simulink model "PSV-based Ventilator Circuit"  (R2016a)
settings: Solver=VariableStepAuto  StartTime=0.0  StopTime=10.0  RelTol=1e-3
undefined symbols (not defined in the file): alfa, cdd, cl, fms, kms, mms, PA, PB, Ps, PT, roh
libraries: sh_lib x5, fl_lib x5
settings Model: Creator=sarim  LastModifiedBy=sarim

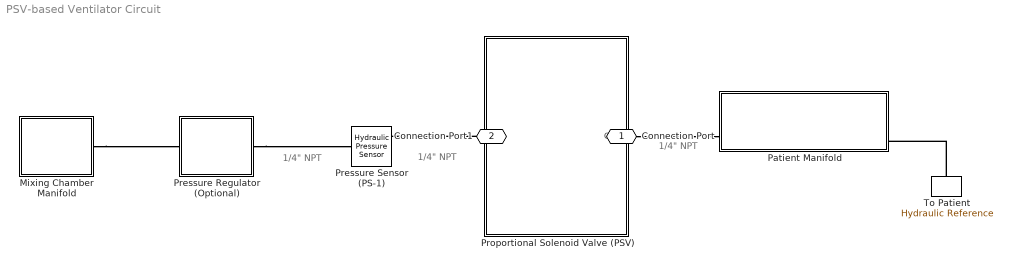
== system PSV-based Ventilator Circuit ==
  note: 1/4" NPT
  note: 1/4" NPT
  note: 1/4" NPT
  Mixing Chamber Manifold : Subsystem
  Patient Manifold : Subsystem
  Pressure Regulator (Optional) : Subsystem
  Pressure Sensor (PS-1) : fl_lib/Hydraulic/Hydraulic Sensors/Hydraulic Pressure Sensor
  Proportional Solenoid Valve (PSV) : Subsystem  VariantControl=Variant1
      mask Display: image('C:\Users\sarim\Desktop\Untitled.png');
  To Patient : fl_lib/Hydraulic/Hydraulic Elements/Hydraulic Reference
  Connection Port : PMIOPort  Port=1  Side=Left
  Connection Port1 : PMIOPort  Port=2  Side=Right
  connections:
  Pressure Regulator (Optional)/RConn1 -- Pressure Sensor (PS-1)/LConn1
  Connection Port1/RConn1 -- Pressure Sensor (PS-1)/RConn1
  Connection Port/RConn1 -- Patient Manifold/LConn2
  To Patient/LConn1 -- Patient Manifold/RConn3
  Mixing Chamber Manifold/RConn1 -- Pressure Regulator (Optional)/LConn1

== system PSV-based Ventilator Circuit/Mixing Chamber Manifold ==
  Air In : PMIOPort  Port=1  Side=Left
  Out : PMIOPort  Port=2  Side=Right
  O2 In : PMIOPort  Port=3  Side=Left

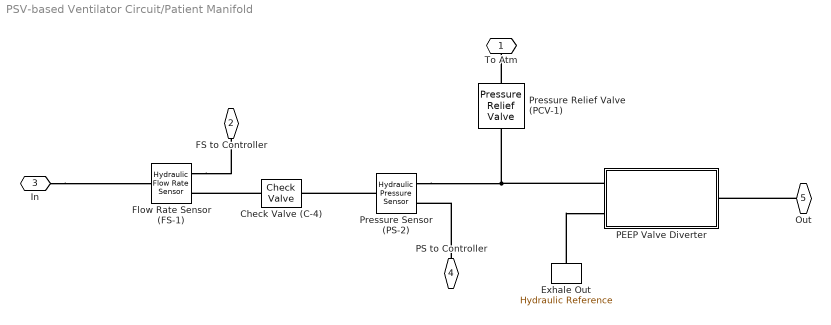
== system PSV-based Ventilator Circuit/Patient Manifold ==
  Check Valve (C-4) : sh_lib/Valves/Directional Valves/Check Valve  area_max=1e-4 m^2  pres_crack=0.3e5 Pa  pres_max=1.2e5 Pa  C_d=0.7  Re_cr=12  A_leak=1e-12 m^2  dynamic=0  tau=0.1 s  area_init=1e-12 m^2
  Exhale Out : fl_lib/Hydraulic/Hydraulic Elements/Hydraulic Reference
  Flow Rate Sensor (FS-1) : fl_lib/Hydraulic/Hydraulic Sensors/Hydraulic Flow Rate Sensor
  PEEP Valve Diverter : Subsystem
  Pressure Sensor (PS-2) : fl_lib/Hydraulic/Hydraulic Sensors/Hydraulic Pressure Sensor
  Pressure Relief Valve (PCV-1) : sh_lib/Valves/Pressure Control Valves/Pressure Relief Valve  area_max=1e-4 m^2  pres_set=50e5 Pa  reg_range=5e5 Pa  C_d=0.7  Re_cr=12  A_leak=1e-12 m^2  dynamic=0  tau=0.1 s  area_init=1e-12 m^2
  To Atm : PMIOPort  Port=1  Side=Left
  FS to Controller : PMIOPort  Port=2  Side=Right
  In : PMIOPort  Port=3  Side=Left
  PS to Controller : PMIOPort  Port=4  Side=Right
  Out : PMIOPort  Port=5  Side=Right
  connections:
  Pressure Relief Valve (PCV-1)/RConn1 -- To Atm/RConn1
  Flow Rate Sensor (FS-1)/RConn1 -- FS to Controller/RConn1
  Exhale Out/LConn1 -- PEEP Valve Diverter/LConn2
  Pressure Sensor (PS-2)/LConn1 -- Check Valve (C-4)/RConn1
  Check Valve (C-4)/LConn1 -- Flow Rate Sensor (FS-1)/RConn2
  In/RConn1 -- Flow Rate Sensor (FS-1)/LConn1
  Pressure Sensor (PS-2)/RConn1 -- PEEP Valve Diverter/LConn1 -- Pressure Relief Valve (PCV-1)/LConn1
  PS to Controller/RConn1 -- Pressure Sensor (PS-2)/RConn2
  Out/RConn1 -- PEEP Valve Diverter/RConn1

== system PSV-based Ventilator Circuit/Pressure Regulator (Optional) ==
  Pressure Reducing Valve : sh_lib/Valves/Pressure Control Valves/Pressure Reducing Valve  area_max=1e-4 m^2  pres_set=5e+6 Pa  reg_range=5e+5 Pa  C_d=0.7  Re_cr=12  A_leak=1e-12 m^2  dynamic=0  tau=0.1 s  area_init=1e-12 m^2
  In : PMIOPort  Port=1  Side=Left
  Out : PMIOPort  Port=2  Side=Right
  connections:
  Pressure Reducing Valve/RConn1 -- Out/RConn1
  Pressure Reducing Valve/LConn1 -- In/RConn1

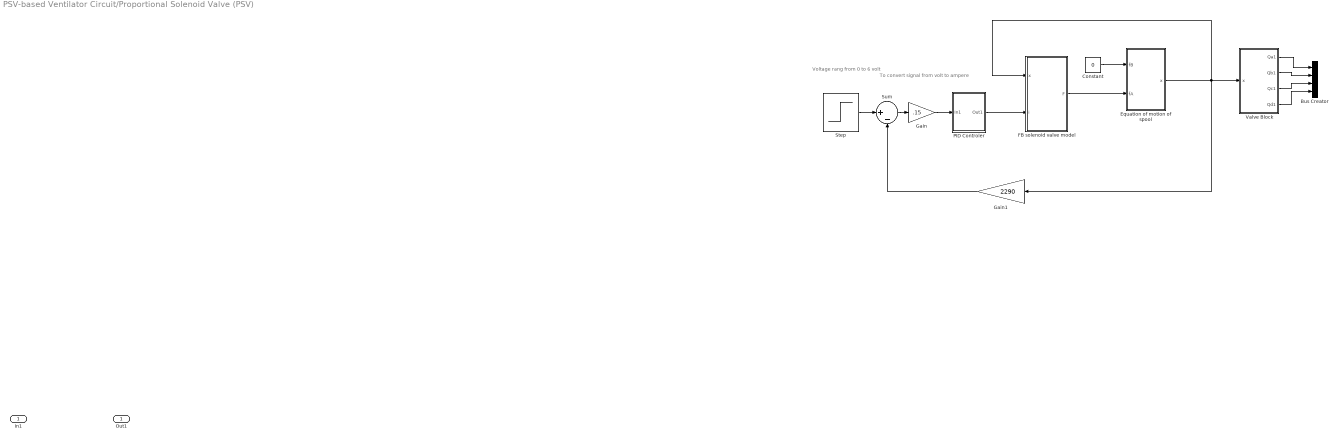
== system PSV-based Ventilator Circuit/Proportional Solenoid Valve (PSV) ==
  note: To convert signal from
      | volt to ampere
  note: Voltage rang
      | from 0 to 6 volt
  In1 : Inport
  Bus Creator : BusCreator  Inputs=4
  Constant : Constant  Value=0
  "Equation of motion of spool " : Subsystem
  FB solenoid valve model : Subsystem
  Gain : Gain  Gain=.15
  Gain1 : Gain  Gain=2290
  PID Controler : Subsystem
  Step : Step  Time=0  After=4.8  SampleTime=0
  Sum : Sum  Inputs=|+-
  Valve Block : Subsystem
  Out1 : Outport
  wires:
  FB solenoid valve model/1(F) -> "Equation of motion of spool "/2(fA)
  Constant/1 -> "Equation of motion of spool "/1(fB)
  Step/1 -> Sum/1
  Sum/1 -> Gain/1
  Gain1/1 -> Sum/2
  PID Controler/1(Out1) -> FB solenoid valve model/2(i)
  Gain/1 -> PID Controler/1(In1)
  "Equation of motion of spool "/1(x) -> Valve Block/1(x), Gain1/1, FB solenoid valve model/1(x)
  Valve Block/1(Qa1) -> Bus Creator/1
  Valve Block/2(Qb1) -> Bus Creator/2
  Valve Block/4(Qd1) -> Bus Creator/4
  Valve Block/3(Qc1) -> Bus Creator/3

== system PSV-based Ventilator Circuit/Patient Manifold/PEEP Valve Diverter ==
  Check Valve1 : sh_lib/Valves/Directional Valves/Check Valve  area_max=1e-4 m^2  pres_crack=0.3e5 Pa  pres_max=1.2e5 Pa  C_d=0.7  Re_cr=12  A_leak=1e-12 m^2  dynamic=0  tau=0.1 s  area_init=1e-12 m^2
  Pressure Relief Valve : sh_lib/Valves/Pressure Control Valves/Pressure Relief Valve  area_max=1e-4 m^2  pres_set=50e5 Pa  reg_range=5e5 Pa  C_d=0.7  Re_cr=12  A_leak=1e-12 m^2  dynamic=0  tau=0.1 s  area_init=1e-12 m^2
  To Patient : PMIOPort  Port=1  Side=Right
  In Line : PMIOPort  Port=2  Side=Left
  Ex Line : PMIOPort  Port=3  Side=Left
  connections:
  Check Valve1/LConn1 -- In Line/RConn1
  To Patient/RConn1 -- Pressure Relief Valve/LConn1 -- Check Valve1/RConn1
  Ex Line/RConn1 -- Pressure Relief Valve/RConn1

== system PSV-based Ventilator Circuit/Proportional Solenoid Valve (PSV)/Equation of motion of spool  ==
  note: x00
  note: x0
  note: x
  note: mms * x00 + fms * x0+ kms *x = fA - fB
  fB : Inport
  fA : Inport  Port=2
  Gain : Gain  Gain=1/mms
  Gain1 : Gain  Gain=kms
  Gain2 : Gain  Gain=fms
  Integrator : Integrator
  Integrator1 : Integrator
  Sum : Sum  Inputs=|+--
  Sum1 : Sum  Inputs=|+-
  x : Outport
  wires:
  Sum/1 -> Gain/1
  Gain/1 -> Integrator/1
  Integrator/1 -> Integrator1/1, Gain2/1
  Integrator1/1 -> Gain1/1, x/1
  Gain2/1 -> Sum/3
  Gain1/1 -> Sum/2
  Sum1/1 -> Sum/1
  fA/1 -> Sum1/1
  fB/1 -> Sum1/2

== system PSV-based Ventilator Circuit/Proportional Solenoid Valve (PSV)/FB solenoid valve model ==
  note: This data from Tamer M. Menshawy
  x : Inport
  i : Inport  Port=2
  Constant1 : Constant  Value=2.5
  Look-Up Table (2-D)2 : Lookup2D  RowIndex=[0.1 0.15 0.2 0.25 0.3 0.35 0.4 0.45 0.5 0.55 0.6 0.65 0.7 0.75 0.8]  ColumnIndex=[1 2 3 4 5]  Table=[0 0 0 0 0; 0 0 0 0 0; 0 0 3.32 5.39 11.27; 0.31 1.65 6.12 11.64 15.98; 1.44 3.06 9.05 17.58 20.43; 2.56 4.23 11.14 21.53 24.09; 4.03 5.41 13.45 25.17 28.62; 5.39 7.12 16.87 28.75 32.52; 6.3 8.74 19.51 32.25 36.91; 7.77 10.31 21.9 35.86 40.36; 8.82 11.95 24.54 39.27 44.63; 9.73 13.81 27.1 43.06 48.68; 11.06 15.54 29.66 46.33 52.61; 12.84 17.58 31.52 49.05 55.75; 14.15 19.85 32.8 51.82 59.93]  SaturateOnIntegerOverflow=on
  Sum2 : Sum  SaturateOnIntegerOverflow=on
  f2 : Gain  Gain=1000  SaturateOnIntegerOverflow=on  OutDataTypeStr=Inherit: Same as input  ParamDataTypeStr=Inherit: Same as input
  F : Outport
  wires:
  i/1 -> Look-Up Table (2-D)2/1
  f2/1 -> Sum2/1
  Constant1/1 -> Sum2/2
  Sum2/1 -> Look-Up Table (2-D)2/2
  x/1 -> f2/1
  Look-Up Table (2-D)2/1 -> F/1

== system PSV-based Ventilator Circuit/Proportional Solenoid Valve (PSV)/PID Controler ==
  note: P
  note: I
  note: D
  In1 : Inport
  Derivative : Derivative
  Gain3 : Gain  Gain=.5
  Gain4 : Gain  Gain=36
  Gain5 : Gain  Gain=0.001
  Integrator : Integrator
  Sum1 : Sum  Inputs=+++
  Out1 : Outport
  wires:
  In1/1 -> Integrator/1, Derivative/1, Gain3/1
  Gain3/1 -> Sum1/1
  Integrator/1 -> Gain4/1
  Gain4/1 -> Sum1/2
  Derivative/1 -> Gain5/1
  Gain5/1 -> Sum1/3
  Sum1/1 -> Out1/1

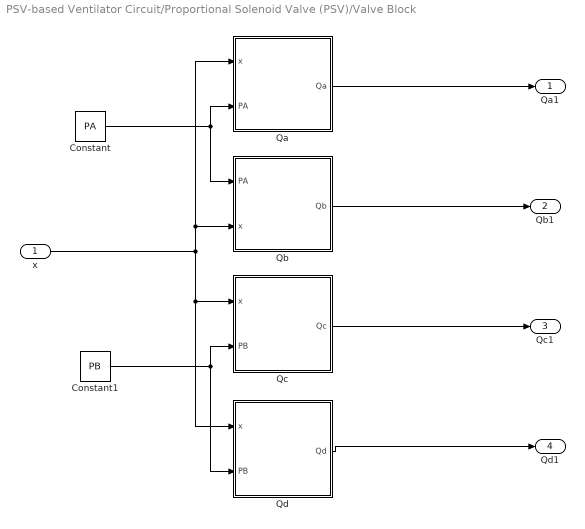
== system PSV-based Ventilator Circuit/Proportional Solenoid Valve (PSV)/Valve Block ==
  x : Inport
  Constant : Constant  Value=PA
  Constant1 : Constant  Value=PB
  Qa : Subsystem
  Qb : Subsystem
  "Qc " : Subsystem
  Qd : Subsystem
  Qa1 : Outport
  Qb1 : Outport  Port=2
  Qc1 : Outport  Port=3
  Qd1 : Outport  Port=4
  wires:
  Qa/1(Qa) -> Qa1/1
  x/1 -> "Qc "/1(x), Qd/1(x), Qb/2(x), Qa/1(x)
  Constant/1 -> Qa/2(PA), Qb/1(PA)
  Qb/1(Qb) -> Qb1/1
  "Qc "/1(Qc) -> Qc1/1
  Qd/1(Qd) -> Qd1/1
  Constant1/1 -> Qd/2(PB), "Qc "/2(PB)

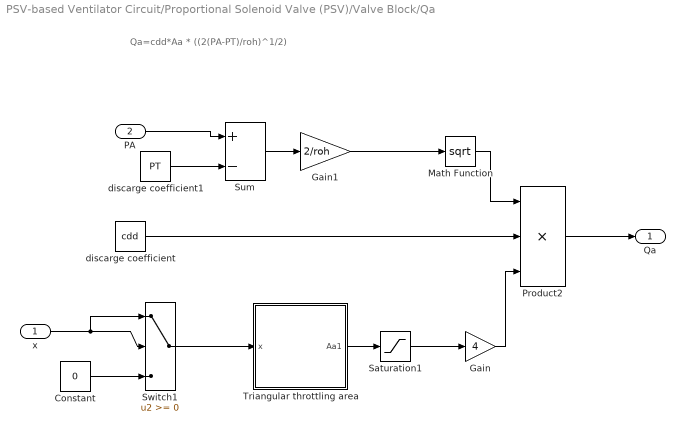
== system PSV-based Ventilator Circuit/Proportional Solenoid Valve (PSV)/Valve Block/Qa ==
  note: Qa=cdd*Aa * ((2(PA-PT)/roh)^1/2)
  x : Inport
  PA : Inport  Port=2
  Constant : Constant  Value=0
  Gain : Gain  Gain=4
  Gain1 : Gain  Gain=2/roh
  Math Function : Math  Operator=sqrt  SaturateOnIntegerOverflow=on
  Product2 : Product  Inputs=3  RndMeth=Zero
  Saturation1 : Saturate  UpperLimit=1  LowerLimit=cl
  Sum : Sum  Inputs=+-
  Switch1 : Switch
  "Triangular throttling area " : Subsystem
  discarge coefficient : Constant  Value=cdd
  discarge coefficient1 : Constant  Value=PT
  Qa : Outport
  wires:
  PA/1 -> Sum/1
  discarge coefficient/1 -> Product2/2
  discarge coefficient1/1 -> Sum/2
  Sum/1 -> Gain1/1
  Gain1/1 -> Math Function/1
  Math Function/1 -> Product2/1
  Product2/1 -> Qa/1
  "Triangular throttling area "/1(Aa1) -> Saturation1/1
  Saturation1/1 -> Gain/1
  Constant/1 -> Switch1/3
  Switch1/1 -> "Triangular throttling area "/1(x)
  x/1 -> Switch1/1, Switch1/2
  Gain/1 -> Product2/3

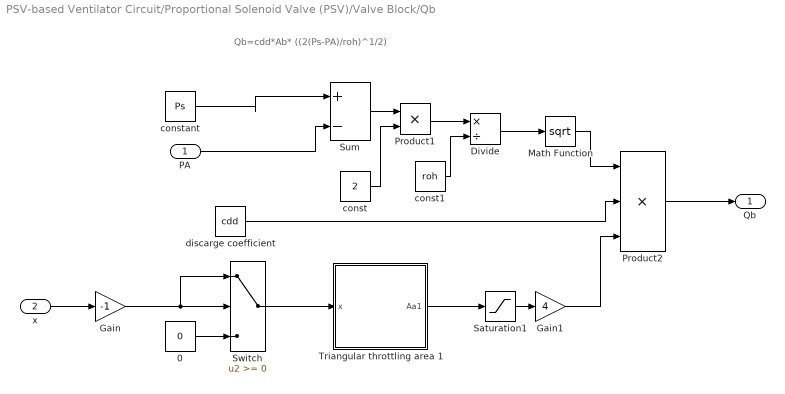
== system PSV-based Ventilator Circuit/Proportional Solenoid Valve (PSV)/Valve Block/Qb ==
  note: Qb=cdd*Ab* ((2(Ps-PA)/roh)^1/2)
  PA : Inport
  x : Inport  Port=2
  0 : Constant  Value=0
  Divide : Product  Inputs=*/
  Gain : Gain  Gain=-1
  Gain1 : Gain  Gain=4
  Math Function : Math  Operator=sqrt  SaturateOnIntegerOverflow=on
  Product1 : Product  RndMeth=Zero
  Product2 : Product  Inputs=3  RndMeth=Zero
  Saturation1 : Saturate  LowerLimit=cl
  Sum : Sum  Inputs=|+-
  Switch : Switch  SaturateOnIntegerOverflow=on
  Triangular throttling area 1 : Subsystem
  const : Constant  Value=2
  const1 : Constant  Value=roh
  constant : Constant  Value=Ps
  discarge coefficient : Constant  Value=cdd
  Qb : Outport
  wires:
  Product2/1 -> Qb/1
  Math Function/1 -> Product2/1
  Divide/1 -> Math Function/1
  const1/1 -> Divide/2
  Product1/1 -> Divide/1
  const/1 -> Product1/2
  Sum/1 -> Product1/1
  discarge coefficient/1 -> Product2/2
  constant/1 -> Sum/1
  PA/1 -> Sum/2
  Triangular throttling area 1/1(Aa1) -> Saturation1/1
  Saturation1/1 -> Gain1/1
  0/1 -> Switch/3
  Switch/1 -> Triangular throttling area 1/1(x)
  x/1 -> Gain/1
  Gain/1 -> Switch/2, Switch/1
  Gain1/1 -> Product2/3

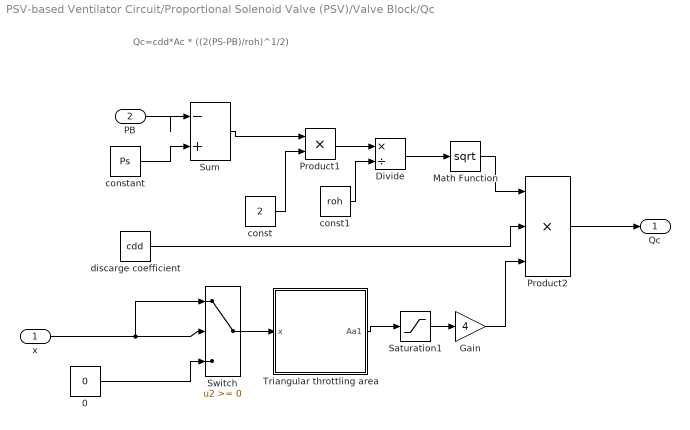
== system PSV-based Ventilator Circuit/Proportional Solenoid Valve (PSV)/Valve Block/Qc  ==
  note: Qc=cdd*Ac * ((2(PS-PB)/roh)^1/2)
  x : Inport
  PB : Inport  Port=2
  0 : Constant  Value=0
  Divide : Product  Inputs=*/
  Gain : Gain  Gain=4
  Math Function : Math  Operator=sqrt  SaturateOnIntegerOverflow=on
  Product1 : Product  RndMeth=Zero
  Product2 : Product  Inputs=3  RndMeth=Zero
  Saturation1 : Saturate  UpperLimit=2  LowerLimit=cl
  Sum : Sum  Inputs=|-+
  Switch : Switch  SaturateOnIntegerOverflow=on
  "Triangular throttling area " : Subsystem
  const : Constant  Value=2
  const1 : Constant  Value=roh
  constant : Constant  Value=Ps
  discarge coefficient : Constant  Value=cdd
  Qc : Outport
  wires:
  discarge coefficient/1 -> Product2/2
  Sum/1 -> Product1/1
  const/1 -> Product1/2
  Product1/1 -> Divide/1
  const1/1 -> Divide/2
  Divide/1 -> Math Function/1
  Math Function/1 -> Product2/1
  Product2/1 -> Qc/1
  PB/1 -> Sum/1
  constant/1 -> Sum/2
  "Triangular throttling area "/1(Aa1) -> Saturation1/1
  Saturation1/1 -> Gain/1
  0/1 -> Switch/3
  x/1 -> Switch/2, Switch/1
  Switch/1 -> "Triangular throttling area "/1(x)
  Gain/1 -> Product2/3

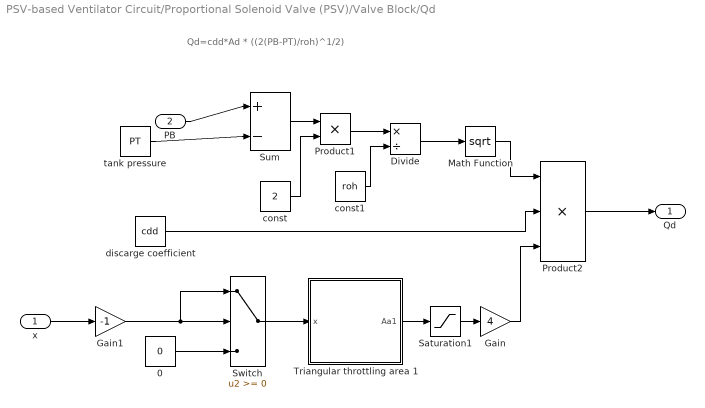
== system PSV-based Ventilator Circuit/Proportional Solenoid Valve (PSV)/Valve Block/Qd ==
  note: Qd=cdd*Ad * ((2(PB-PT)/roh)^1/2)
  x : Inport
  PB : Inport  Port=2
  0 : Constant  Value=0
  Divide : Product  Inputs=*/
  Gain : Gain  Gain=4
  Gain1 : Gain  Gain=-1
  Math Function : Math  Operator=sqrt  SaturateOnIntegerOverflow=on
  Product1 : Product  RndMeth=Zero
  Product2 : Product  Inputs=3  RndMeth=Zero
  Saturation1 : Saturate  LowerLimit=cl
  Sum : Sum  Inputs=|+-
  Switch : Switch  SaturateOnIntegerOverflow=on
  Triangular throttling area 1 : Subsystem
  const : Constant  Value=2
  const1 : Constant  Value=roh
  discarge coefficient : Constant  Value=cdd
  tank pressure : Constant  Value=PT
  Qd : Outport
  wires:
  discarge coefficient/1 -> Product2/2
  Sum/1 -> Product1/1
  const/1 -> Product1/2
  Product1/1 -> Divide/1
  const1/1 -> Divide/2
  Divide/1 -> Math Function/1
  Math Function/1 -> Product2/1
  Product2/1 -> Qd/1
  Triangular throttling area 1/1(Aa1) -> Saturation1/1
  Saturation1/1 -> Gain/1
  x/1 -> Gain1/1
  Gain1/1 -> Switch/2, Switch/1
  Switch/1 -> Triangular throttling area 1/1(x)
  Gain/1 -> Product2/3
  tank pressure/1 -> Sum/2
  PB/1 -> Sum/1
  0/1 -> Switch/3

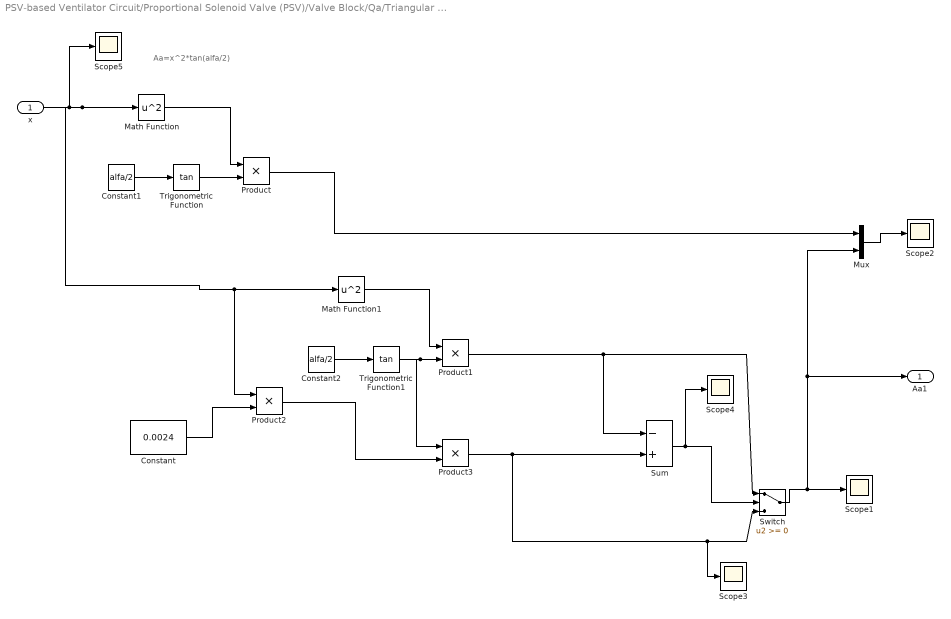
== system PSV-based Ventilator Circuit/Proportional Solenoid Valve (PSV)/Valve Block/Qa/Triangular throttling area  ==
  note: Aa=x^2*tan(alfa/2)
  x : Inport
  Constant : Constant  Value=0.0024
  Constant1 : Constant  Value=alfa/2
  Constant2 : Constant  Value=alfa/2
  Math Function : Math  Operator=square  SaturateOnIntegerOverflow=on
  Math Function1 : Math  Operator=square  SaturateOnIntegerOverflow=on
  Mux : Mux  Inputs=2
  Product{,1..3} (4 alike) : Product  RndMeth=Zero
  Scope{1..5} (5 alike) : Scope
  Sum : Sum  Inputs=-+
  Switch : Switch
  Trigonometric Function : Trigonometry  Operator=tan
  Trigonometric Function1 : Trigonometry  Operator=tan
  Aa1 : Outport
  wires:
  Constant1/1 -> Trigonometric Function/1
  Trigonometric Function/1 -> Product/2
  Math Function/1 -> Product/1
  x/1 -> Math Function/1, Math Function1/1, Product2/1, Scope5/1
  Product/1 -> Mux/1
  Constant2/1 -> Trigonometric Function1/1
  Trigonometric Function1/1 -> Product1/2, Product3/1
  Math Function1/1 -> Product1/1
  Product1/1 -> Switch/1, Sum/1
  Constant/1 -> Product2/2
  Product2/1 -> Product3/2
  Product3/1 -> Sum/2, Switch/3, Scope3/1
  Sum/1 -> Switch/2, Scope4/1
  Switch/1 -> Scope1/1, Aa1/1, Mux/2
  Mux/1 -> Scope2/1

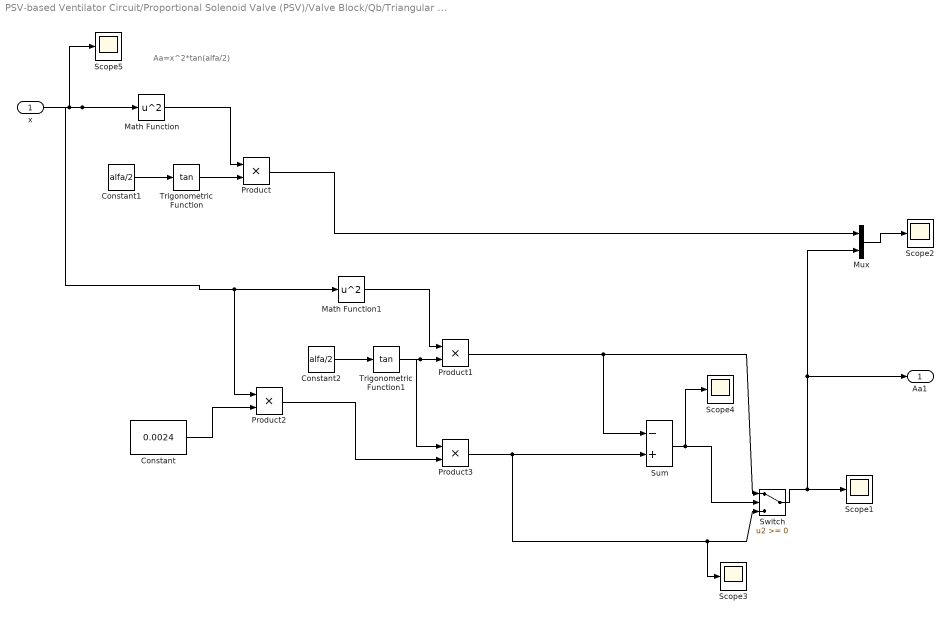
== system PSV-based Ventilator Circuit/Proportional Solenoid Valve (PSV)/Valve Block/Qb/Triangular throttling area 1 ==
  note: Aa=x^2*tan(alfa/2)
  x : Inport
  Constant : Constant  Value=0.0024
  Constant1 : Constant  Value=alfa/2
  Constant2 : Constant  Value=alfa/2
  Math Function : Math  Operator=square  SaturateOnIntegerOverflow=on
  Math Function1 : Math  Operator=square  SaturateOnIntegerOverflow=on
  Mux : Mux  Inputs=2
  Product{,1..3} (4 alike) : Product  RndMeth=Zero
  Scope{1..5} (5 alike) : Scope
  Sum : Sum  Inputs=-+
  Switch : Switch
  Trigonometric Function : Trigonometry  Operator=tan
  Trigonometric Function1 : Trigonometry  Operator=tan
  Aa1 : Outport
  wires:
  Constant1/1 -> Trigonometric Function/1
  Trigonometric Function/1 -> Product/2
  Math Function/1 -> Product/1
  x/1 -> Math Function/1, Math Function1/1, Product2/1, Scope5/1
  Product/1 -> Mux/1
  Constant2/1 -> Trigonometric Function1/1
  Trigonometric Function1/1 -> Product1/2, Product3/1
  Math Function1/1 -> Product1/1
  Product1/1 -> Switch/1, Sum/1
  Constant/1 -> Product2/2
  Product2/1 -> Product3/2
  Product3/1 -> Sum/2, Switch/3, Scope3/1
  Sum/1 -> Switch/2, Scope4/1
  Switch/1 -> Scope1/1, Aa1/1, Mux/2
  Mux/1 -> Scope2/1

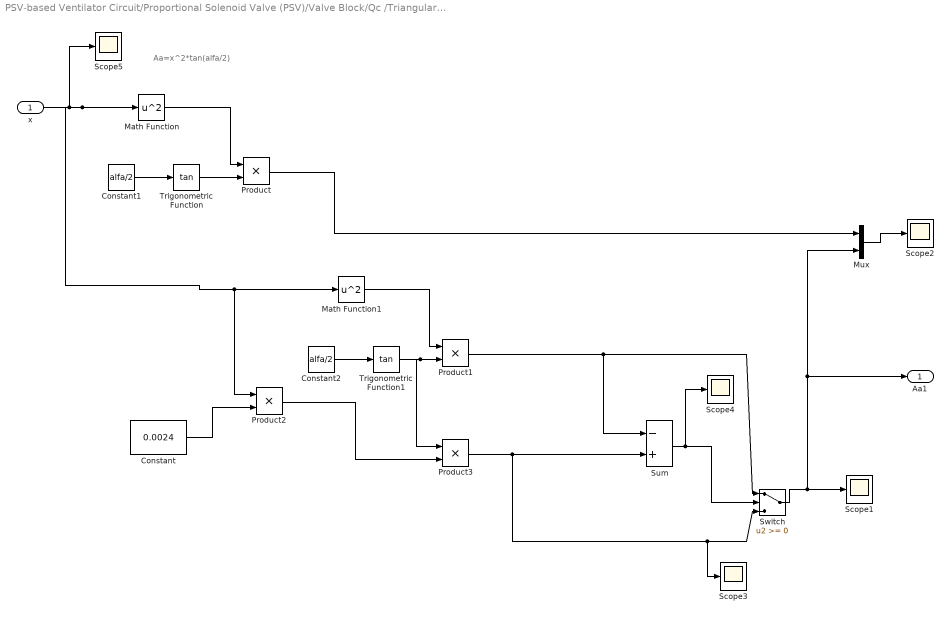
== system PSV-based Ventilator Circuit/Proportional Solenoid Valve (PSV)/Valve Block/Qc /Triangular throttling area  ==
  note: Aa=x^2*tan(alfa/2)
  x : Inport
  Constant : Constant  Value=0.0024
  Constant1 : Constant  Value=alfa/2
  Constant2 : Constant  Value=alfa/2
  Math Function : Math  Operator=square  SaturateOnIntegerOverflow=on
  Math Function1 : Math  Operator=square  SaturateOnIntegerOverflow=on
  Mux : Mux  Inputs=2
  Product{,1..3} (4 alike) : Product  RndMeth=Zero
  Scope{1..5} (5 alike) : Scope
  Sum : Sum  Inputs=-+
  Switch : Switch
  Trigonometric Function : Trigonometry  Operator=tan
  Trigonometric Function1 : Trigonometry  Operator=tan
  Aa1 : Outport
  wires:
  Constant1/1 -> Trigonometric Function/1
  Trigonometric Function/1 -> Product/2
  Math Function/1 -> Product/1
  x/1 -> Math Function/1, Math Function1/1, Product2/1, Scope5/1
  Product/1 -> Mux/1
  Constant2/1 -> Trigonometric Function1/1
  Trigonometric Function1/1 -> Product1/2, Product3/1
  Math Function1/1 -> Product1/1
  Product1/1 -> Switch/1, Sum/1
  Constant/1 -> Product2/2
  Product2/1 -> Product3/2
  Product3/1 -> Sum/2, Switch/3, Scope3/1
  Sum/1 -> Switch/2, Scope4/1
  Switch/1 -> Scope1/1, Aa1/1, Mux/2
  Mux/1 -> Scope2/1

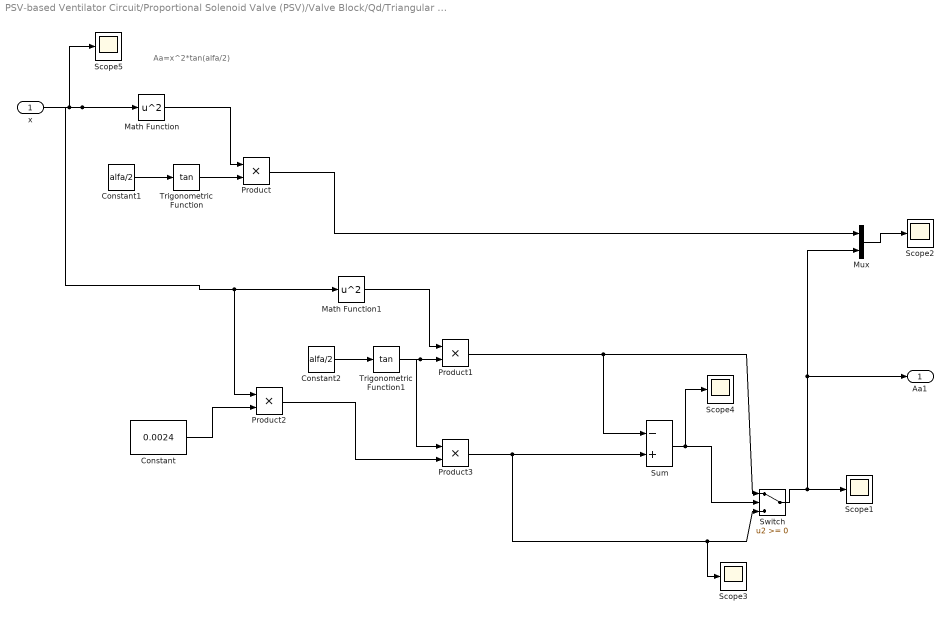
== system PSV-based Ventilator Circuit/Proportional Solenoid Valve (PSV)/Valve Block/Qd/Triangular throttling area 1 ==
  note: Aa=x^2*tan(alfa/2)
  x : Inport
  Constant : Constant  Value=0.0024
  Constant1 : Constant  Value=alfa/2
  Constant2 : Constant  Value=alfa/2
  Math Function : Math  Operator=square  SaturateOnIntegerOverflow=on
  Math Function1 : Math  Operator=square  SaturateOnIntegerOverflow=on
  Mux : Mux  Inputs=2
  Product{,1..3} (4 alike) : Product  RndMeth=Zero
  Scope{1..5} (5 alike) : Scope
  Sum : Sum  Inputs=-+
  Switch : Switch
  Trigonometric Function : Trigonometry  Operator=tan
  Trigonometric Function1 : Trigonometry  Operator=tan
  Aa1 : Outport
  wires:
  Constant1/1 -> Trigonometric Function/1
  Trigonometric Function/1 -> Product/2
  Math Function/1 -> Product/1
  x/1 -> Math Function/1, Math Function1/1, Product2/1, Scope5/1
  Product/1 -> Mux/1
  Constant2/1 -> Trigonometric Function1/1
  Trigonometric Function1/1 -> Product1/2, Product3/1
  Math Function1/1 -> Product1/1
  Product1/1 -> Switch/1, Sum/1
  Constant/1 -> Product2/2
  Product2/1 -> Product3/2
  Product3/1 -> Sum/2, Switch/3, Scope3/1
  Sum/1 -> Switch/2, Scope4/1
  Switch/1 -> Scope1/1, Aa1/1, Mux/2
  Mux/1 -> Scope2/1
